simulink library "monroe_library"  (R2012b)
settings: Solver=ode45  StartTime=0.0  StopTime=10.0  RelTol=1e-3
values from neighbouring files (symbols this model uses):
  input_bit_width = ', num2str(input_bit_width))    [fft_direct_draw.m]
undefined symbols (not defined in the file or in its folder): gcbh, xlBlockLoadCallback
libraries: xbsIndex_r4 x1880, monroe_library x159, casper_library x13, xps_library x1
(part 23 of 43)

== system monroe_library/direct_coeff_gen/coeff_gen_stage_3_group_2 ==
  sync : Inport
  Concat : xbsIndex_r4/Concat  num_inputs=2  dbl_ovrd=off  block_type=concat
  Concat1 : xbsIndex_r4/Concat  num_inputs=2  dbl_ovrd=off  block_type=concat
  Concat2 : xbsIndex_r4/Concat  num_inputs=2  dbl_ovrd=off  block_type=concat
  Constant : xbsIndex_r4/Constant  arith_type=Boolean  const=0  n_bits=16  bin_pt=14  explicit_period=on  period=1  equ=P=C  opselect=C  inp2=PCIN>>17  opr=+  inp1=P  carry=CIN  dbl_ovrd=off  block_type=constant
  Constant1 : xbsIndex_r4/Constant  arith_type=Boolean  const=1  n_bits=16  bin_pt=14  explicit_period=off  period=1  equ=P=C  opselect=C  inp2=PCIN>>17  opr=+  inp1=P  carry=CIN  dbl_ovrd=off  block_type=constant
  Constant3 : xbsIndex_r4/Constant  arith_type=Signed (2's comp)  const=0  n_bits=18  bin_pt=17  explicit_period=on  period=1  equ=P=C  opselect=C  inp2=PCIN>>17  opr=+  inp1=P  carry=CIN  dbl_ovrd=off  block_type=constant
  Constant4 : xbsIndex_r4/Constant  arith_type=Boolean  const=0  n_bits=16  bin_pt=14  explicit_period=off  period=1  equ=P=C  opselect=C  inp2=PCIN>>17  opr=+  inp1=P  carry=CIN  dbl_ovrd=off  block_type=constant
  Constant5 : xbsIndex_r4/Constant  arith_type=Unsigned  const=2  n_bits=10  bin_pt=0  explicit_period=on  period=1  equ=P=C  opselect=C  inp2=PCIN>>17  opr=+  inp1=P  carry=CIN  dbl_ovrd=off  block_type=constant
  Counter : xbsIndex_r4/Counter  cnt_type=Free Running  cnt_to=Inf  operation=Up  start_count=0  cnt_by_val=1  arith_type=Unsigned  n_bits=10  bin_pt=0  load_pin=on  rst=off  en=off  explicit_period=on  period=1  dbl_ovrd=off  use_behavioral_HDL=off  implementation=Fabric  block_type=counter
  Delay : xbsIndex_r4/Delay  en=off  latency=0  dbl_ovrd=off  reg_retiming=off  block_type=delay
  Dual Port RAM4 : xbsIndex_r4/Dual Port RAM  depth=2048  initVector=[-1 -0.999999705862882 -0.999998823451702 -0.999997352766978 -0.999995293809576 -0.999992646580707 -0.999989411081928 -0.999985587315143 -0.999981175282601 -0.999976174986898 -0.999970586430974 -0.999964409618118 -0.999957644551964 -0.99995029123649 -0.999942349676024 -0.999933819875236 -0.999924701839145 -0.999914995573113 -0.999904701082853 -0.999893818374418 -0.999882347454213 -0.999870288328983 -0.999857641005824 -0.999844405492175 -0.999830581795823 -0.9998161699249 -0.999801169887884 -0.999785581693599 -0.999769405351215 -0.999752640870249 -0.999735288260562 -0.999717347532362 -0.999698818696204 -0.999679701762988 -0.999659996743959 -0.99963970365071 -0.999618822495179 -0.999597353289648 -0.999575296046749 -0.999552650779457 -0.999529417501093 -0.999505596225325 -0.999481186966167 -0.999456189737977 -0.999430604555462 -0.999404431433671 -0.999377670388003 -0.999350321434199 -0.99932238458835 -0.999293859866888 -0.999264747286594 -0.999235046864596 -0.999204758618364 -0.999173882565716 -0.999142418724817 -0.999110367114175 -0.999077727752645 -0.999044500659429 -0.999010685854073 -0.99897628335647 -0.998941293186857 -0.998905715365818 -0.998869549914284 -0.998832796853528 -0.998795456205172 -0.998757527991183 -0.998719012233873 -0.998679908955899 -0.998640218180265 -0.99859993993032 -0.998559074229759 -0.998517621102622 -0.998475580573295 -0.998432952666508 -0.99838973740734 -0.998345934821212 -0.998301544933893 -0.998256567771495 -0.998211003360478 -0.998164851727646 -0.998118112900149 -0.998070786905482 -0.998022873771486 -0.997974373526347 -0.997925286198596 -0.99787561181711 -0.997825350411112 -0.997774502010168 -0.997723066644192 -0.997671044343441 -0.99761843513852 -0.997565239060376 -0.997511456140303 -0.997457086409942 -0.997402129901275 -0.997346586646633 -0.99729045667869 -0.997233740030466 -0.997176436735326 -0.99711854682698 -0.997060070339483 -0.997001007307235 -0.996941357764982 -0.996881121747814 -0.996820299291166 -0.996758890430818 -0.996696895202896 -0.99663431364387 -0.996571145790555 -0.996507391680111 -0.996443051350043 -0.9963781248382 -0.996312612182778 -0.996246513422316 -0.996179828595697 -0.996112557742151 -0.996044700901252 -0.995976258112918 -0.995907229417412 -0.995837614855342 -0.99576741446766 -0.995696628295664 -0.995625256380994 -0.995553298765639 -0.995480755491927 -0.995407626602535 -0.995333912140482 -0.995259612149133 -0.995184726672197 -0.995109255753726 -0.995033199438119 -0.994956557770116 -0.994879330794806 -0.994801518557617 -0.994723121104326 -0.994644138481051 -0.994564570734255 -0.994484417910748 -0.994403680057679 -0.994322357222546 -0.994240449453188 -0.99415795679779 -0.994074879304879 -0.993991217023329 -0.993906970002356 -0.99382213829152 -0.993736721940725 -0.993650721000219 -0.993564135520595 -0.993476965552789 -0.993389211148081 -0.993300872358093 -0.993211949234795 -0.993122441830496 -0.993032350197851 -0.99294167438986 -0.992850414459865 -0.992758570461551 -0.992666142448948 -0.992573130476429 -0.99247953459871 -0.992385354870852 -0.992290591348257 -0.992195244086674 -0.992099313142192 -0.992002798571245 -0.991905700430609 -0.991808018777407 -0.9917097536691 -0.991610905163495 -0.991511473318744 -0.991411458193339 -0.991310859846115 -0.991209678336254 -0.991107913723277 -0.991005566067049 -0.99090263542778 -0.99079912186602 -0.990695025442665 -0.99059034621895 -0.990485084256457 -0.990379239617108 -0.990272812363169 -0.990165802557248 -0.990058210262297 -0.989950035541609 -0.989841278458821 -0.989731939077911 -0.989622017463201 -0.989511513679355 -0.98940042779138 -0.989288759864625 -0.989176509964781 -0.989063678157882 -0.988950264510303 -0.988836269088764 -0.988721691960324 -0.988606533192387 -0.988490792852697 -0.988374471009341 -0.988257567730749 -0.988140083085693 -0.988022017143284 -0.987903369972978 -0.987784141644572 -0.987664332228206 -0.987543941794359 -0.987422970413855 -0.987301418157858 -0.987179285097874 -0.987056571305751 -0.986933276853678 ...(+34809 chars)]  distributed_mem=Block RAM  init_a=0  init_b=0  rst_a=off  rst_b=off  en_a=off  en_b=off  latency=2  write_mode_A=No Read On Write  write_mode_B=No Read On Write  dbl_ovrd=off  optimize=Area  use_rpm=on  block_type=dpram
  Reinterpret : xbsIndex_r4/Reinterpret  force_arith_type=on  arith_type=Unsigned  force_bin_pt=on  bin_pt=0  block_type=reinterpret
      settings: infoedit="Changes signal type without altering the binary representation.   You can changed the signal between signed and unsigned, and relocate the binary point.<br><br>Hardware notes: In hardware this block costs nothing.<br><br>Example:  Suppose the input is 6 bits wide, signed, with 2 fractional bits, and the output is forced to unsigned with 0 fractional bits.  Then an input of -2.0 (1110.00 in binary 2's complement) becomes an output of 56 (111000 in binary)."
  Reinterpret1 : xbsIndex_r4/Reinterpret  force_arith_type=on  arith_type=Unsigned  force_bin_pt=on  bin_pt=0  block_type=reinterpret
      settings: infoedit="Changes signal type without altering the binary representation.   You can changed the signal between signed and unsigned, and relocate the binary point.<br><br>Hardware notes: In hardware this block costs nothing.<br><br>Example:  Suppose the input is 6 bits wide, signed, with 2 fractional bits, and the output is forced to unsigned with 0 fractional bits.  Then an input of -2.0 (1110.00 in binary 2's complement) becomes an output of 56 (111000 in binary)."
  count_slice : xbsIndex_r4/Slice  nbits=10  boolean_output=off  mode=Upper Bit Location + Width  bit1=0  base1=MSB of Input  bit0=0  base0=MSB of Input  dbl_ovrd=off  block_type=slice
  coeff : Outport
  wires:
  count_slice/1 -> Concat1/2, Concat/2  "xlsub2_Counter_out1"
  Constant3/1 -> Dual Port RAM4/5, Dual Port RAM4/2  "xlsub2_Constant3_out1"
  Constant/1 -> Dual Port RAM4/6, Dual Port RAM4/3  "xlsub2_Constant_out1"
  Reinterpret1/1 -> Concat2/2  "xlsub2_Reinterpret1_out1"
  Dual Port RAM4/2 -> Reinterpret1/1  "xlsub2_Dual_Port_RAM4_out2"
  Reinterpret/1 -> Concat2/1  "xlsub2_Reinterpret_out1"
  Dual Port RAM4/1 -> Reinterpret/1  "xlsub2_Dual_Port_RAM4_out1"
  Concat1/1 -> Dual Port RAM4/4  "xlsub2_Concat1_out1"
  Concat/1 -> Dual Port RAM4/1  "xlsub2_Concat_out1"
  Delay/1 -> coeff/1
  Concat2/1 -> Delay/1  "xlsub2_Concat2_out1"
  Counter/1 -> count_slice/1
  Constant5/1 -> Counter/2  "xlsub2_Constant5_out1"
  sync/1 -> Counter/1
  Constant4/1 -> Concat1/1  "xlsub2_Constant4_out1"
  Constant1/1 -> Concat/1  "xlsub2_Constant1_out1"
